simulink model "CPG_for_4Leg"  (Simulink 8.0)
settings: Solver=ode23t  StartTime=0.0  StopTime=10  MaxStep=1e-3  RelTol=1e-3
undefined symbols (not defined in the file): alpha, amp, cw_FL_HL, cw_FR_FL, cw_FR_HR, cw_HR_HL, FL_HL_lag, FR_FL_lag, FR_HR_lag, freq, HR_HL_lag, tau
settings Model: Creator=Metti  LastModifiedBy=Metti
settings SolverCC: ZeroCrossControl=DisableAll
settings DataIOCC: SignalLoggingSaveFormat=ModelDataLogs
settings DebuggingCC: FcnCallInpInsideContextMsg=EnableAllAsWarning
settings ConfigurationSet: Description=SimMechanics 2G

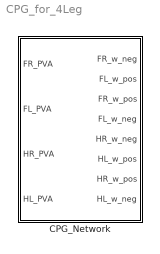
== system CPG_for_4Leg ==
  CPG_Network : Subsystem

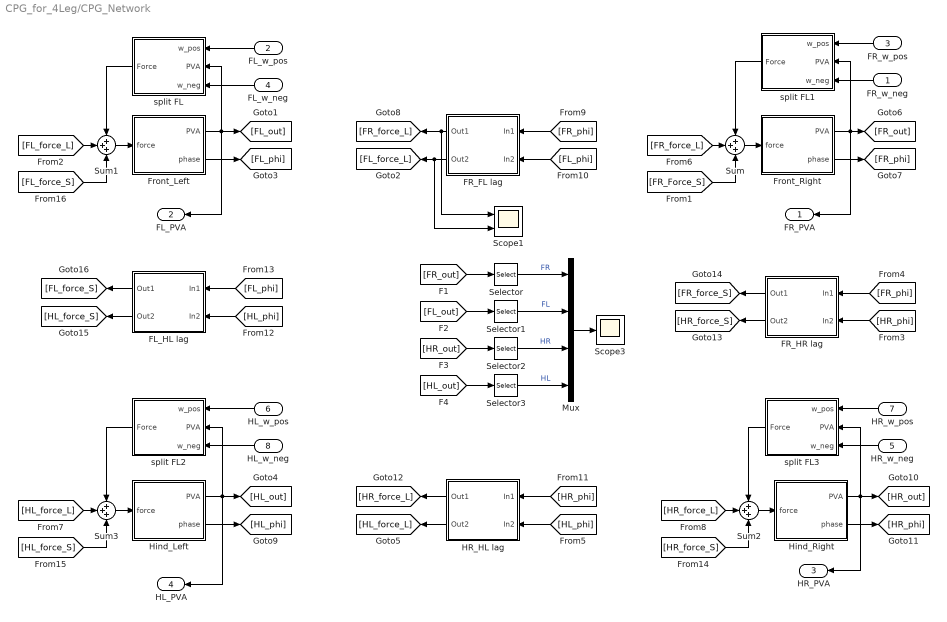
== system CPG_for_4Leg/CPG_Network ==
  FR_w_neg : Inport
  FL_w_pos : Inport  Port=2
  FR_w_pos : Inport  Port=3
  FL_w_neg : Inport  Port=4
  HR_w_neg : Inport  Port=5
  HL_w_pos : Inport  Port=6
  HR_w_pos : Inport  Port=7
  HL_w_neg : Inport  Port=8
  FL_HL lag : Subsystem  mask{d_phase=FL_HL_lag, coupling_weight=cw_FL_HL}
      mask prompts: d_phase "Phase Lag"; coupling_weight "Coupling Weight"
  FR_FL lag : Subsystem  mask{d_phase=FR_FL_lag, coupling_weight=cw_FR_FL}
      mask prompts: d_phase "Phase Lag"; coupling_weight "Coupling Weight"
  FR_HR lag : Subsystem  mask{d_phase=FR_HR_lag, coupling_weight=cw_FR_HR}
      mask prompts: d_phase "Phase Lag"; coupling_weight "Coupling Weight"
  Front_Left : Subsystem  mask{Amp=amp, Offset=0, init_phi=0}
      mask prompts: Amp "Amplitude"; init_phi "Initial Phase"
  Front_Right : Subsystem  mask{Amp=amp, Offset=0, init_phi=0}
      mask prompts: Amp "Amplitude"; init_phi "Initial Phase"
  HR_HL lag : Subsystem  mask{d_phase=HR_HL_lag, coupling_weight=cw_HR_HL}
      mask prompts: d_phase "Phase Lag"; coupling_weight "Coupling Weight"
  Hind_Left : Subsystem  mask{Amp=amp, Offset=0, init_phi=0}
      mask prompts: Amp "Amplitude"; init_phi "Initial Phase"
  Hind_Right : Subsystem  mask{Amp=amp, Offset=0, init_phi=0}
      mask prompts: Amp "Amplitude"; init_phi "Initial Phase"
  Mux : Mux
  Scope1 : Scope  NumInputPorts=2
      settings: ShowLegends=on  TimeRange=10  YMin=0~-5  YMax=2~5  SaveName=Output1
  Scope3 : Scope
      settings: ShowLegends=on  TimeRange=10  YMin=0  YMax=2  SaveName=Output
  Selector{,1..3} (4 alike) : Selector  InputPortWidth=3  IndexOptions=Index vector (dialog)  Indices=[1]  OutputSizes=1
  Sum{,1..3} (4 alike) : Sum  Inputs=+++
  split FL : Subsystem
  split FL1 : Subsystem
  split FL2 : Subsystem
  split FL3 : Subsystem
  FR_PVA : Outport
  FL_PVA : Outport  Port=2
  HR_PVA : Outport  Port=3
  HL_PVA : Outport  Port=4
  wires:
  Mux/1 -> Scope3/1
  Front_Left/2(phase) -> [FL_phi]
  Front_Right/2(phase) -> [FR_phi]
  [FL_phi] -> FR_FL lag/2(In2)
  [FR_phi] -> FR_FL lag/1(In1)
  FR_FL lag/1(Out1) -> Scope1/1, [FR_force_L]
  FR_FL lag/2(Out2) -> Scope1/2, [FL_force_L]
  Front_Right/1(PVA) -> split FL1/2(PVA), FR_PVA/1, [FR_out]
  [FL_force_L] -> Sum1/2
  Sum1/1 -> Front_Left/1(force)
  Sum/1 -> Front_Right/1(force)
  [FR_force_L] -> Sum/2
  [FL_out] -> Selector1/1
  Selector1/1 -> Mux/2  "FL"
  Selector/1 -> Mux/1  "FR"
  [FR_out] -> Selector/1
  FR_w_pos/1 -> split FL1/1(w_pos)
  FR_w_neg/1 -> split FL1/3(w_neg)
  split FL1/1(Force) -> Sum/1
  FL_w_pos/1 -> split FL/1(w_pos)
  FL_w_neg/1 -> split FL/3(w_neg)
  Front_Left/1(PVA) -> split FL/2(PVA), FL_PVA/1, [FL_out]
  split FL/1(Force) -> Sum1/1
  Hind_Left/2(phase) -> [HL_phi]
  Hind_Right/2(phase) -> [HR_phi]
  [HL_phi] -> HR_HL lag/2(In2)
  [HR_phi] -> HR_HL lag/1(In1)
  HR_HL lag/1(Out1) -> [HR_force_L]
  HR_HL lag/2(Out2) -> [HL_force_L]
  Hind_Right/1(PVA) -> split FL3/2(PVA), HR_PVA/1, [HR_out]
  [HL_force_L] -> Sum3/2
  Sum3/1 -> Hind_Left/1(force)
  Sum2/1 -> Hind_Right/1(force)
  [HR_force_L] -> Sum2/2
  HR_w_pos/1 -> split FL3/1(w_pos)
  HR_w_neg/1 -> split FL3/3(w_neg)
  split FL3/1(Force) -> Sum2/1
  HL_w_pos/1 -> split FL2/1(w_pos)
  HL_w_neg/1 -> split FL2/3(w_neg)
  Hind_Left/1(PVA) -> split FL2/2(PVA), HL_PVA/1, [HL_out]
  split FL2/1(Force) -> Sum3/1
  [HR_phi] -> FR_HR lag/2(In2)
  [FR_phi] -> FR_HR lag/1(In1)
  FR_HR lag/1(Out1) -> [FR_force_S]
  FR_HR lag/2(Out2) -> [HR_force_S]
  [HL_phi] -> FL_HL lag/2(In2)
  [FL_phi] -> FL_HL lag/1(In1)
  FL_HL lag/1(Out1) -> [FL_force_S]
  FL_HL lag/2(Out2) -> [HL_force_S]
  [HL_out] -> Selector3/1
  Selector3/1 -> Mux/4  "HL"
  Selector2/1 -> Mux/3  "HR"
  [HR_out] -> Selector2/1
  [FR_Force_S] -> Sum/3
  [HR_force_S] -> Sum2/3
  [HL_force_S] -> Sum3/3
  [FL_force_S] -> Sum1/3

== system CPG_for_4Leg/CPG_Network/FL_HL lag ==
  In1 : Inport
  In2 : Inport  Port=2
  Constant : Constant  Value=d_phase
  Gain : Gain  Gain=-1
  Sum : Sum  Inputs=--+
  sin : Fcn  Expr=coupling_weight*sin(u(1))
  Out1 : Outport
  Out2 : Outport  Port=2
  wires:
  Sum/1 -> sin/1
  sin/1 -> Gain/1, Out1/1
  Constant/1 -> Sum/2
  In1/1 -> Sum/1
  In2/1 -> Sum/3
  Gain/1 -> Out2/1

== system CPG_for_4Leg/CPG_Network/FR_FL lag ==
  In1 : Inport
  In2 : Inport  Port=2
  Constant : Constant  Value=d_phase
  Gain : Gain  Gain=-1
  Sum : Sum  Inputs=--+
  sin : Fcn  Expr=coupling_weight*sin(u(1))
  Out1 : Outport
  Out2 : Outport  Port=2
  wires:
  Sum/1 -> sin/1
  sin/1 -> Gain/1, Out1/1
  Constant/1 -> Sum/2
  In1/1 -> Sum/1
  In2/1 -> Sum/3
  Gain/1 -> Out2/1

== system CPG_for_4Leg/CPG_Network/FR_HR lag ==
  In1 : Inport
  In2 : Inport  Port=2
  Constant : Constant  Value=d_phase
  Gain : Gain  Gain=-1
  Sum : Sum  Inputs=--+
  sin : Fcn  Expr=coupling_weight*sin(u(1))
  Out1 : Outport
  Out2 : Outport  Port=2
  wires:
  Gain/1 -> Out2/1
  In2/1 -> Sum/3
  In1/1 -> Sum/1
  Constant/1 -> Sum/2
  sin/1 -> Out1/1, Gain/1
  Sum/1 -> sin/1

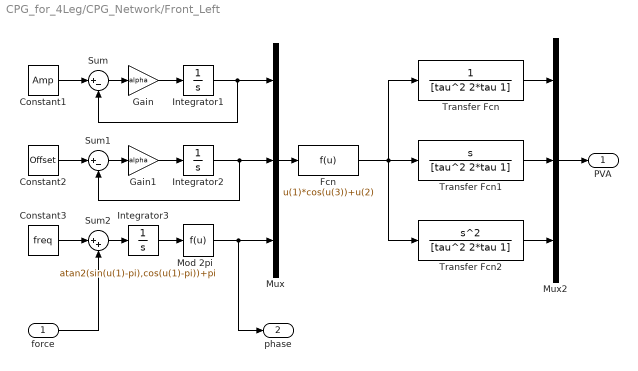
== system CPG_for_4Leg/CPG_Network/Front_Left ==
  force : Inport
  Constant1 : Constant  Value=Amp
  Constant2 : Constant  Value=Offset
  Constant3 : Constant  Value=freq
  Fcn : Fcn  Expr=u(1)*cos(u(3))+u(2)
  Gain : Gain  Gain=alpha
  Gain1 : Gain  Gain=alpha
  Integrator1 : Integrator
  Integrator2 : Integrator
  Integrator3 : Integrator  InitialCondition=init_phi + 0.01*rand
  Mod 2pi : Fcn  Expr=atan2(sin(u(1)-pi),cos(u(1)-pi))+pi
  Mux : Mux  Inputs=3
  Mux2 : Mux  Inputs=3
  Sum : Sum  Inputs=|+-
  Sum1 : Sum  Inputs=|+-
  Sum2 : Sum  Inputs=|++
  Transfer Fcn : TransferFcn  Denominator=[tau^2 2*tau 1]
  Transfer Fcn1 : TransferFcn  Numerator=[1 0]  Denominator=[tau^2 2*tau 1]
  Transfer Fcn2 : TransferFcn  Numerator=[1 0 0]  Denominator=[tau^2 2*tau 1]
  PVA : Outport
  phase : Outport  Port=2
  wires:
  Mux2/1 -> PVA/1
  Fcn/1 -> Transfer Fcn1/1, Transfer Fcn/1, Transfer Fcn2/1
  Transfer Fcn1/1 -> Mux2/2
  Transfer Fcn/1 -> Mux2/1
  Transfer Fcn2/1 -> Mux2/3
  force/1 -> Sum2/2
  Sum2/1 -> Integrator3/1
  Constant3/1 -> Sum2/1
  Integrator3/1 -> Mod 2pi/1
  Mod 2pi/1 -> Mux/3, phase/1
  Mux/1 -> Fcn/1
  Gain1/1 -> Integrator2/1
  Constant2/1 -> Sum1/1
  Integrator2/1 -> Mux/2, Sum1/2
  Sum1/1 -> Gain1/1
  Gain/1 -> Integrator1/1
  Constant1/1 -> Sum/1
  Integrator1/1 -> Mux/1, Sum/2
  Sum/1 -> Gain/1

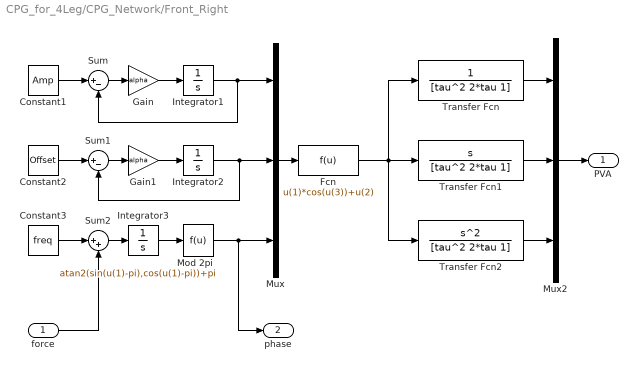
== system CPG_for_4Leg/CPG_Network/Front_Right ==
  force : Inport
  Constant1 : Constant  Value=Amp
  Constant2 : Constant  Value=Offset
  Constant3 : Constant  Value=freq
  Fcn : Fcn  Expr=u(1)*cos(u(3))+u(2)
  Gain : Gain  Gain=alpha
  Gain1 : Gain  Gain=alpha
  Integrator1 : Integrator
  Integrator2 : Integrator
  Integrator3 : Integrator  InitialCondition=init_phi + 0.01*rand
  Mod 2pi : Fcn  Expr=atan2(sin(u(1)-pi),cos(u(1)-pi))+pi
  Mux : Mux  Inputs=3
  Mux2 : Mux  Inputs=3
  Sum : Sum  Inputs=|+-
  Sum1 : Sum  Inputs=|+-
  Sum2 : Sum  Inputs=|++
  Transfer Fcn : TransferFcn  Denominator=[tau^2 2*tau 1]
  Transfer Fcn1 : TransferFcn  Numerator=[1 0]  Denominator=[tau^2 2*tau 1]
  Transfer Fcn2 : TransferFcn  Numerator=[1 0 0]  Denominator=[tau^2 2*tau 1]
  PVA : Outport
  phase : Outport  Port=2
  wires:
  Sum/1 -> Gain/1
  Integrator1/1 -> Sum/2, Mux/1
  Constant1/1 -> Sum/1
  Gain/1 -> Integrator1/1
  Sum1/1 -> Gain1/1
  Integrator2/1 -> Sum1/2, Mux/2
  Constant2/1 -> Sum1/1
  Gain1/1 -> Integrator2/1
  Mux/1 -> Fcn/1
  Mod 2pi/1 -> phase/1, Mux/3
  Integrator3/1 -> Mod 2pi/1
  Constant3/1 -> Sum2/1
  Sum2/1 -> Integrator3/1
  force/1 -> Sum2/2
  Transfer Fcn2/1 -> Mux2/3
  Transfer Fcn/1 -> Mux2/1
  Transfer Fcn1/1 -> Mux2/2
  Fcn/1 -> Transfer Fcn2/1, Transfer Fcn/1, Transfer Fcn1/1
  Mux2/1 -> PVA/1

== system CPG_for_4Leg/CPG_Network/HR_HL lag ==
  In1 : Inport
  In2 : Inport  Port=2
  Constant : Constant  Value=d_phase
  Gain : Gain  Gain=-1
  Sum : Sum  Inputs=--+
  sin : Fcn  Expr=coupling_weight*sin(u(1))
  Out1 : Outport
  Out2 : Outport  Port=2
  wires:
  Gain/1 -> Out2/1
  In2/1 -> Sum/3
  In1/1 -> Sum/1
  Constant/1 -> Sum/2
  sin/1 -> Out1/1, Gain/1
  Sum/1 -> sin/1

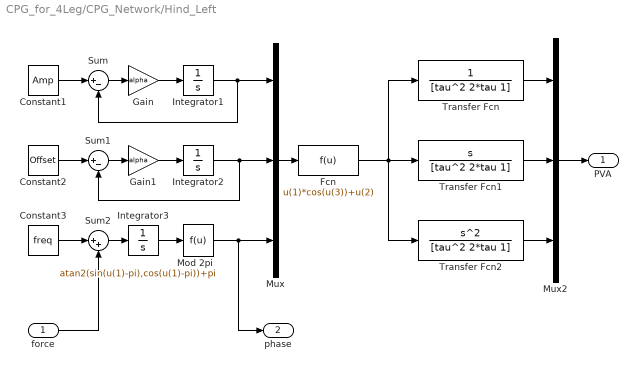
== system CPG_for_4Leg/CPG_Network/Hind_Left ==
  force : Inport
  Constant1 : Constant  Value=Amp
  Constant2 : Constant  Value=Offset
  Constant3 : Constant  Value=freq
  Fcn : Fcn  Expr=u(1)*cos(u(3))+u(2)
  Gain : Gain  Gain=alpha
  Gain1 : Gain  Gain=alpha
  Integrator1 : Integrator
  Integrator2 : Integrator
  Integrator3 : Integrator  InitialCondition=init_phi + 0.01*rand
  Mod 2pi : Fcn  Expr=atan2(sin(u(1)-pi),cos(u(1)-pi))+pi
  Mux : Mux  Inputs=3
  Mux2 : Mux  Inputs=3
  Sum : Sum  Inputs=|+-
  Sum1 : Sum  Inputs=|+-
  Sum2 : Sum  Inputs=|++
  Transfer Fcn : TransferFcn  Denominator=[tau^2 2*tau 1]
  Transfer Fcn1 : TransferFcn  Numerator=[1 0]  Denominator=[tau^2 2*tau 1]
  Transfer Fcn2 : TransferFcn  Numerator=[1 0 0]  Denominator=[tau^2 2*tau 1]
  PVA : Outport
  phase : Outport  Port=2
  wires:
  Sum/1 -> Gain/1
  Integrator1/1 -> Sum/2, Mux/1
  Constant1/1 -> Sum/1
  Gain/1 -> Integrator1/1
  Sum1/1 -> Gain1/1
  Integrator2/1 -> Sum1/2, Mux/2
  Constant2/1 -> Sum1/1
  Gain1/1 -> Integrator2/1
  Mux/1 -> Fcn/1
  Mod 2pi/1 -> phase/1, Mux/3
  Integrator3/1 -> Mod 2pi/1
  Constant3/1 -> Sum2/1
  Sum2/1 -> Integrator3/1
  force/1 -> Sum2/2
  Transfer Fcn2/1 -> Mux2/3
  Transfer Fcn/1 -> Mux2/1
  Transfer Fcn1/1 -> Mux2/2
  Fcn/1 -> Transfer Fcn2/1, Transfer Fcn/1, Transfer Fcn1/1
  Mux2/1 -> PVA/1

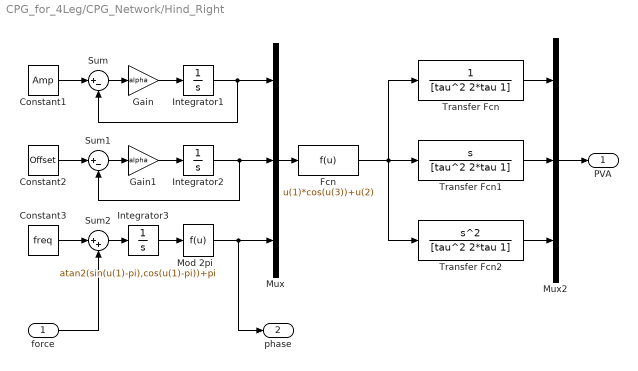
== system CPG_for_4Leg/CPG_Network/Hind_Right ==
  force : Inport
  Constant1 : Constant  Value=Amp
  Constant2 : Constant  Value=Offset
  Constant3 : Constant  Value=freq
  Fcn : Fcn  Expr=u(1)*cos(u(3))+u(2)
  Gain : Gain  Gain=alpha
  Gain1 : Gain  Gain=alpha
  Integrator1 : Integrator
  Integrator2 : Integrator
  Integrator3 : Integrator  InitialCondition=init_phi + 0.01*rand
  Mod 2pi : Fcn  Expr=atan2(sin(u(1)-pi),cos(u(1)-pi))+pi
  Mux : Mux  Inputs=3
  Mux2 : Mux  Inputs=3
  Sum : Sum  Inputs=|+-
  Sum1 : Sum  Inputs=|+-
  Sum2 : Sum  Inputs=|++
  Transfer Fcn : TransferFcn  Denominator=[tau^2 2*tau 1]
  Transfer Fcn1 : TransferFcn  Numerator=[1 0]  Denominator=[tau^2 2*tau 1]
  Transfer Fcn2 : TransferFcn  Numerator=[1 0 0]  Denominator=[tau^2 2*tau 1]
  PVA : Outport
  phase : Outport  Port=2
  wires:
  Mux2/1 -> PVA/1
  Fcn/1 -> Transfer Fcn1/1, Transfer Fcn/1, Transfer Fcn2/1
  Transfer Fcn1/1 -> Mux2/2
  Transfer Fcn/1 -> Mux2/1
  Transfer Fcn2/1 -> Mux2/3
  force/1 -> Sum2/2
  Sum2/1 -> Integrator3/1
  Constant3/1 -> Sum2/1
  Integrator3/1 -> Mod 2pi/1
  Mod 2pi/1 -> Mux/3, phase/1
  Mux/1 -> Fcn/1
  Gain1/1 -> Integrator2/1
  Constant2/1 -> Sum1/1
  Integrator2/1 -> Mux/2, Sum1/2
  Sum1/1 -> Gain1/1
  Gain/1 -> Integrator1/1
  Constant1/1 -> Sum/1
  Integrator1/1 -> Mux/1, Sum/2
  Sum/1 -> Gain/1

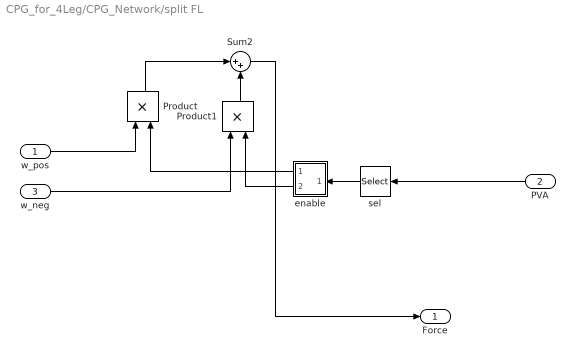
== system CPG_for_4Leg/CPG_Network/split FL ==
  w_pos : Inport
  PVA : Inport  Port=2
  w_neg : Inport  Port=3
  Product : Product  RndMeth=Zero
  Product1 : Product  RndMeth=Zero
  Sum2 : Sum  Inputs=|++
  enable : Subsystem
  sel : Selector  InputPortWidth=3  IndexOptions=Index vector (dialog)  Indices=[2]  OutputSizes=1
  Force : Outport
  wires:
  Product/1 -> Sum2/1
  w_pos/1 -> Product/1
  w_neg/1 -> Product1/1
  Product1/1 -> Sum2/2
  PVA/1 -> sel/1
  enable/1(pos) -> Product/2
  enable/2(neg) -> Product1/2
  Sum2/1 -> Force/1
  sel/1 -> enable/1(in)

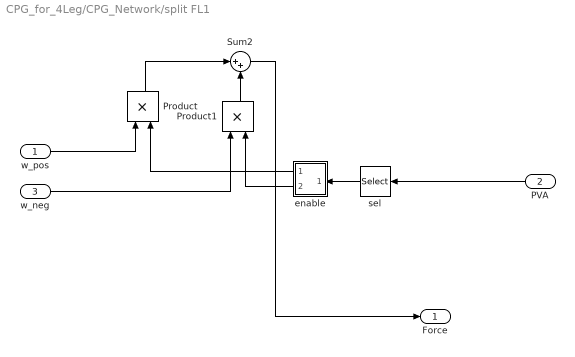
== system CPG_for_4Leg/CPG_Network/split FL1 ==
  w_pos : Inport
  PVA : Inport  Port=2
  w_neg : Inport  Port=3
  Product : Product  RndMeth=Zero
  Product1 : Product  RndMeth=Zero
  Sum2 : Sum  Inputs=|++
  enable : Subsystem
  sel : Selector  InputPortWidth=3  IndexOptions=Index vector (dialog)  Indices=[2]  OutputSizes=1
  Force : Outport
  wires:
  sel/1 -> enable/1(in)
  Sum2/1 -> Force/1
  enable/2(neg) -> Product1/2
  enable/1(pos) -> Product/2
  PVA/1 -> sel/1
  Product1/1 -> Sum2/2
  w_neg/1 -> Product1/1
  w_pos/1 -> Product/1
  Product/1 -> Sum2/1

== system CPG_for_4Leg/CPG_Network/split FL2 ==
  w_pos : Inport
  PVA : Inport  Port=2
  w_neg : Inport  Port=3
  Product : Product  RndMeth=Zero
  Product1 : Product  RndMeth=Zero
  Sum2 : Sum  Inputs=|++
  enable : Subsystem
  sel : Selector  InputPortWidth=3  IndexOptions=Index vector (dialog)  Indices=[2]  OutputSizes=1
  Force : Outport
  wires:
  Product/1 -> Sum2/1
  w_pos/1 -> Product/1
  w_neg/1 -> Product1/1
  Product1/1 -> Sum2/2
  PVA/1 -> sel/1
  enable/1(pos) -> Product/2
  enable/2(neg) -> Product1/2
  Sum2/1 -> Force/1
  sel/1 -> enable/1(in)

== system CPG_for_4Leg/CPG_Network/split FL3 ==
  w_pos : Inport
  PVA : Inport  Port=2
  w_neg : Inport  Port=3
  Product : Product  RndMeth=Zero
  Product1 : Product  RndMeth=Zero
  Sum2 : Sum  Inputs=|++
  enable : Subsystem
  sel : Selector  InputPortWidth=3  IndexOptions=Index vector (dialog)  Indices=[2]  OutputSizes=1
  Force : Outport
  wires:
  Product/1 -> Sum2/1
  w_pos/1 -> Product/1
  w_neg/1 -> Product1/1
  Product1/1 -> Sum2/2
  PVA/1 -> sel/1
  enable/1(pos) -> Product/2
  enable/2(neg) -> Product1/2
  Sum2/1 -> Force/1
  sel/1 -> enable/1(in)

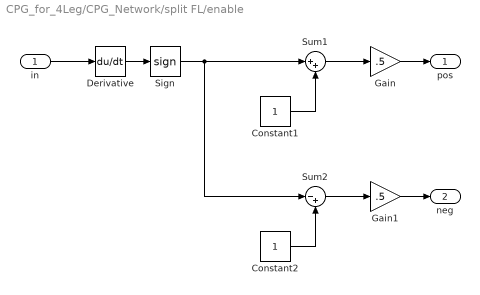
== system CPG_for_4Leg/CPG_Network/split FL/enable ==
  in : Inport
  Constant1 : Constant
  Constant2 : Constant
  Derivative : Derivative
  Gain : Gain  Gain=.5
  Gain1 : Gain  Gain=.5
  Sign : Signum
  Sum1 : Sum  Inputs=|++
  Sum2 : Sum  Inputs=|-+
  pos : Outport
  neg : Outport  Port=2
  wires:
  Derivative/1 -> Sign/1
  Constant1/1 -> Sum1/2
  Sign/1 -> Sum2/1, Sum1/1
  Gain/1 -> pos/1
  in/1 -> Derivative/1
  Sum1/1 -> Gain/1
  Constant2/1 -> Sum2/2
  Gain1/1 -> neg/1
  Sum2/1 -> Gain1/1

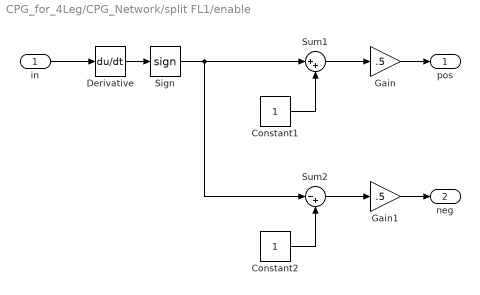
== system CPG_for_4Leg/CPG_Network/split FL1/enable ==
  in : Inport
  Constant1 : Constant
  Constant2 : Constant
  Derivative : Derivative
  Gain : Gain  Gain=.5
  Gain1 : Gain  Gain=.5
  Sign : Signum
  Sum1 : Sum  Inputs=|++
  Sum2 : Sum  Inputs=|-+
  pos : Outport
  neg : Outport  Port=2
  wires:
  Sum2/1 -> Gain1/1
  Gain1/1 -> neg/1
  Constant2/1 -> Sum2/2
  Sum1/1 -> Gain/1
  in/1 -> Derivative/1
  Gain/1 -> pos/1
  Sign/1 -> Sum1/1, Sum2/1
  Constant1/1 -> Sum1/2
  Derivative/1 -> Sign/1

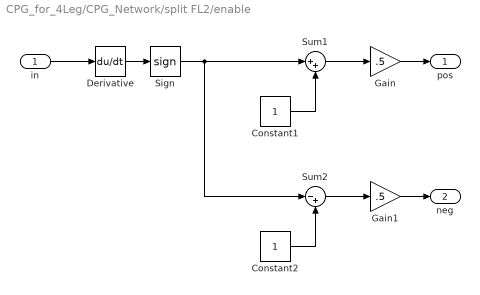
== system CPG_for_4Leg/CPG_Network/split FL2/enable ==
  in : Inport
  Constant1 : Constant
  Constant2 : Constant
  Derivative : Derivative
  Gain : Gain  Gain=.5
  Gain1 : Gain  Gain=.5
  Sign : Signum
  Sum1 : Sum  Inputs=|++
  Sum2 : Sum  Inputs=|-+
  pos : Outport
  neg : Outport  Port=2
  wires:
  Derivative/1 -> Sign/1
  Constant1/1 -> Sum1/2
  Sign/1 -> Sum2/1, Sum1/1
  Gain/1 -> pos/1
  in/1 -> Derivative/1
  Sum1/1 -> Gain/1
  Constant2/1 -> Sum2/2
  Gain1/1 -> neg/1
  Sum2/1 -> Gain1/1

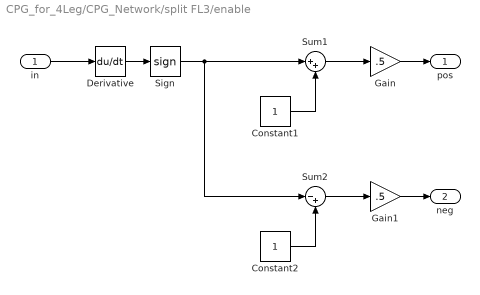
== system CPG_for_4Leg/CPG_Network/split FL3/enable ==
  in : Inport
  Constant1 : Constant
  Constant2 : Constant
  Derivative : Derivative
  Gain : Gain  Gain=.5
  Gain1 : Gain  Gain=.5
  Sign : Signum
  Sum1 : Sum  Inputs=|++
  Sum2 : Sum  Inputs=|-+
  pos : Outport
  neg : Outport  Port=2
  wires:
  Derivative/1 -> Sign/1
  Constant1/1 -> Sum1/2
  Sign/1 -> Sum2/1, Sum1/1
  Gain/1 -> pos/1
  in/1 -> Derivative/1
  Sum1/1 -> Gain/1
  Constant2/1 -> Sum2/2
  Gain1/1 -> neg/1
  Sum2/1 -> Gain1/1
